simulink model "busCreators01volt"  (R2025b)
settings: Solver=VariableStepAuto  StartTime=0.0  StopTime=10.0  RelTol=1e-3
settings Model: Creator=gdudgeon  LastModifiedBy=gdudgeon
settings RTWCC: GPUComputeCapability=3.5

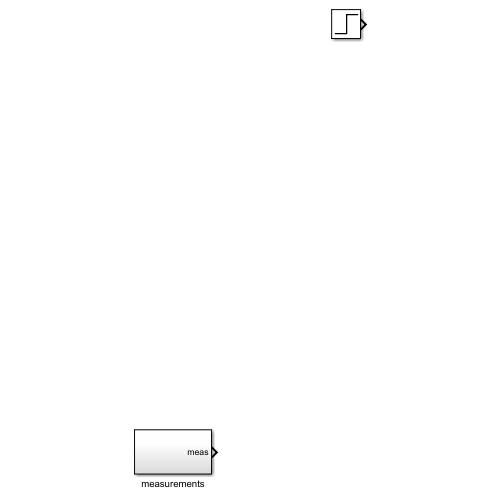
[thumbnail: Simulink's stored preview of the top-level diagram]
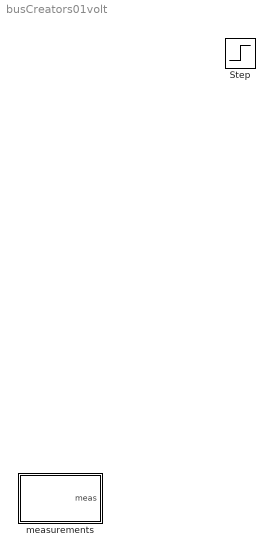
== system busCreators01volt ==
  Step : Step  SampleTime=0
  measurements : Subsystem

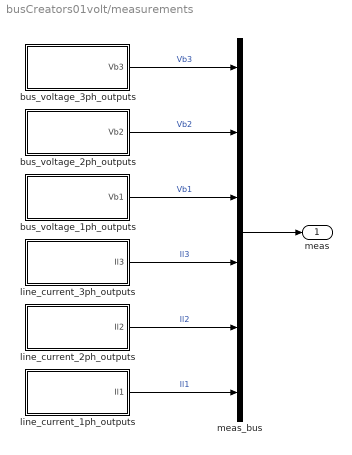
== system busCreators01volt/measurements ==
  bus_voltage_1ph_outputs : Subsystem
  bus_voltage_2ph_outputs : Subsystem
  bus_voltage_3ph_outputs : Subsystem
  line_current_1ph_outputs : Subsystem
  line_current_2ph_outputs : Subsystem
  line_current_3ph_outputs : Subsystem
  meas_bus : BusCreator  Inputs=6
  meas : Outport
  wires:
  line_current_1ph_outputs/1(Il1) -> meas_bus/6  "Il1"
  line_current_2ph_outputs/1(Il2) -> meas_bus/5  "Il2"
  line_current_3ph_outputs/1(Il3) -> meas_bus/4  "Il3"
  meas_bus/1 -> meas/1
  bus_voltage_2ph_outputs/1(Vb2) -> meas_bus/2  "Vb2"
  bus_voltage_3ph_outputs/1(Vb3) -> meas_bus/1  "Vb3"
  bus_voltage_1ph_outputs/1(Vb1) -> meas_bus/3  "Vb1"

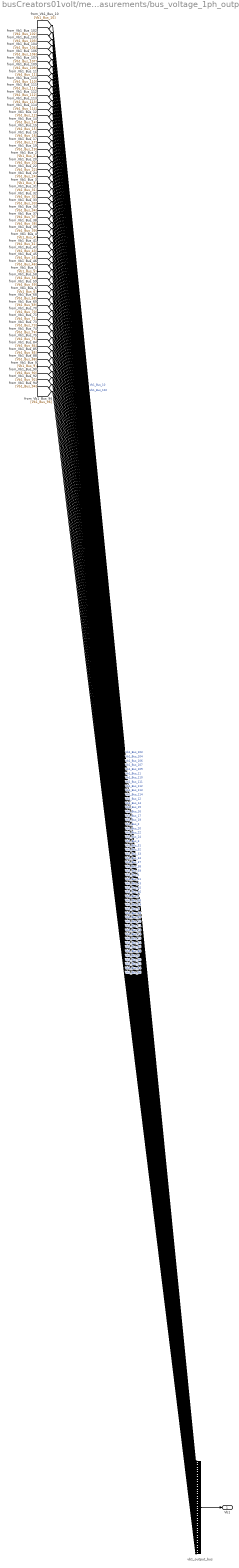
== system busCreators01volt/measurements/bus_voltage_1ph_outputs ==
  vb1_output_bus : BusCreator  Inputs=55
  Vb1 : Outport  OutDataTypeStr=Bus: n1_slBus3  VectorParamsAs1DForOutWhenUnconnected=off
  wires:
  [Vb1_Bus_96] -> vb1_output_bus/55  "Vb1_Bus_96"
  [Vb1_Bus_94] -> vb1_output_bus/54  "Vb1_Bus_94"
  [Vb1_Bus_92] -> vb1_output_bus/53  "Vb1_Bus_92"
  [Vb1_Bus_90] -> vb1_output_bus/52  "Vb1_Bus_90"
  [Vb1_Bus_9] -> vb1_output_bus/51  "Vb1_Bus_9"
  [Vb1_Bus_88] -> vb1_output_bus/50  "Vb1_Bus_88"
  [Vb1_Bus_85] -> vb1_output_bus/49  "Vb1_Bus_85"
  [Vb1_Bus_84] -> vb1_output_bus/48  "Vb1_Bus_84"
  [Vb1_Bus_75] -> vb1_output_bus/47  "Vb1_Bus_75"
  [Vb1_Bus_74] -> vb1_output_bus/46  "Vb1_Bus_74"
  [Vb1_Bus_73] -> vb1_output_bus/45  "Vb1_Bus_73"
  [Vb1_Bus_71] -> vb1_output_bus/44  "Vb1_Bus_71"
  [Vb1_Bus_70] -> vb1_output_bus/43  "Vb1_Bus_70"
  [Vb1_Bus_69] -> vb1_output_bus/42  "Vb1_Bus_69"
  [Vb1_Bus_68] -> vb1_output_bus/41  "Vb1_Bus_68"
  [Vb1_Bus_6] -> vb1_output_bus/40  "Vb1_Bus_6"
  [Vb1_Bus_59] -> vb1_output_bus/39  "Vb1_Bus_59"
  [Vb1_Bus_58] -> vb1_output_bus/38  "Vb1_Bus_58"
  [Vb1_Bus_5] -> vb1_output_bus/37  "Vb1_Bus_5"
  [Vb1_Bus_46] -> vb1_output_bus/36  "Vb1_Bus_46"
  [Vb1_Bus_45] -> vb1_output_bus/35  "Vb1_Bus_45"
  [Vb1_Bus_43] -> vb1_output_bus/34  "Vb1_Bus_43"
  [Vb1_Bus_41] -> vb1_output_bus/33  "Vb1_Bus_41"
  [Vb1_Bus_4] -> vb1_output_bus/32  "Vb1_Bus_4"
  [Vb1_Bus_39] -> vb1_output_bus/31  "Vb1_Bus_39"
  [Vb1_Bus_38] -> vb1_output_bus/30  "Vb1_Bus_38"
  [Vb1_Bus_37] -> vb1_output_bus/29  "Vb1_Bus_37"
  [Vb1_Bus_34] -> vb1_output_bus/28  "Vb1_Bus_34"
  [Vb1_Bus_33] -> vb1_output_bus/27  "Vb1_Bus_33"
  [Vb1_Bus_32] -> vb1_output_bus/26  "Vb1_Bus_32"
  [Vb1_Bus_31] -> vb1_output_bus/25  "Vb1_Bus_31"
  [Vb1_Bus_3] -> vb1_output_bus/24  "Vb1_Bus_3"
  [Vb1_Bus_24] -> vb1_output_bus/23  "Vb1_Bus_24"
  [Vb1_Bus_22] -> vb1_output_bus/22  "Vb1_Bus_22"
  [Vb1_Bus_20] -> vb1_output_bus/21  "Vb1_Bus_20"
  [Vb1_Bus_2] -> vb1_output_bus/20  "Vb1_Bus_2"
  [Vb1_Bus_19] -> vb1_output_bus/19  "Vb1_Bus_19"
  [Vb1_Bus_17] -> vb1_output_bus/18  "Vb1_Bus_17"
  [Vb1_Bus_16] -> vb1_output_bus/17  "Vb1_Bus_16"
  [Vb1_Bus_15] -> vb1_output_bus/16  "Vb1_Bus_15"
  [Vb1_Bus_14] -> vb1_output_bus/15  "Vb1_Bus_14"
  [Vb1_Bus_12] -> vb1_output_bus/14  "Vb1_Bus_12"
  [Vb1_Bus_114] -> vb1_output_bus/13  "Vb1_Bus_114"
  [Vb1_Bus_113] -> vb1_output_bus/12  "Vb1_Bus_113"
  [Vb1_Bus_112] -> vb1_output_bus/11  "Vb1_Bus_112"
  [Vb1_Bus_111] -> vb1_output_bus/10  "Vb1_Bus_111"
  [Vb1_Bus_110] -> vb1_output_bus/9  "Vb1_Bus_110"
  [Vb1_Bus_11] -> vb1_output_bus/8  "Vb1_Bus_11"
  [Vb1_Bus_109] -> vb1_output_bus/7  "Vb1_Bus_109"
  [Vb1_Bus_107] -> vb1_output_bus/6  "Vb1_Bus_107"
  [Vb1_Bus_106] -> vb1_output_bus/5  "Vb1_Bus_106"
  [Vb1_Bus_104] -> vb1_output_bus/4  "Vb1_Bus_104"
  [Vb1_Bus_103] -> vb1_output_bus/3  "Vb1_Bus_103"
  [Vb1_Bus_102] -> vb1_output_bus/2  "Vb1_Bus_102"
  [Vb1_Bus_10] -> vb1_output_bus/1  "Vb1_Bus_10"
  vb1_output_bus/1 -> Vb1/1

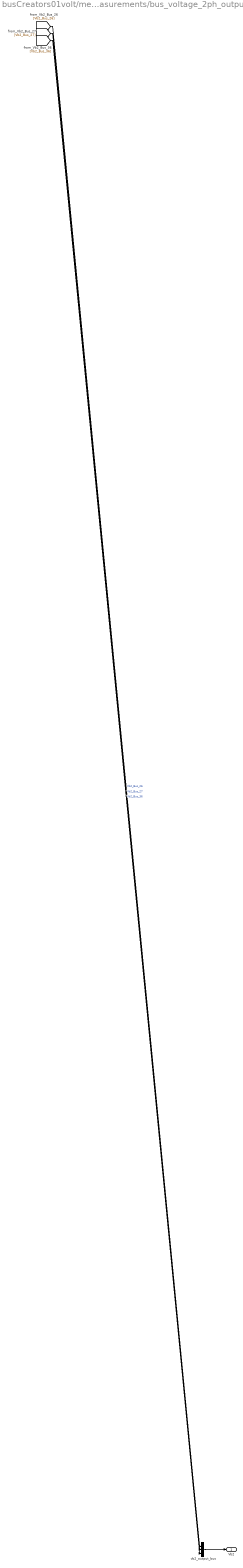
== system busCreators01volt/measurements/bus_voltage_2ph_outputs ==
  vb2_output_bus : BusCreator  Inputs=3
  Vb2 : Outport  OutDataTypeStr=Bus: n1_slBus2  VectorParamsAs1DForOutWhenUnconnected=off
  wires:
  [Vb2_Bus_36] -> vb2_output_bus/3  "Vb2_Bus_36"
  [Vb2_Bus_27] -> vb2_output_bus/2  "Vb2_Bus_27"
  [Vb2_Bus_26] -> vb2_output_bus/1  "Vb2_Bus_26"
  vb2_output_bus/1 -> Vb2/1

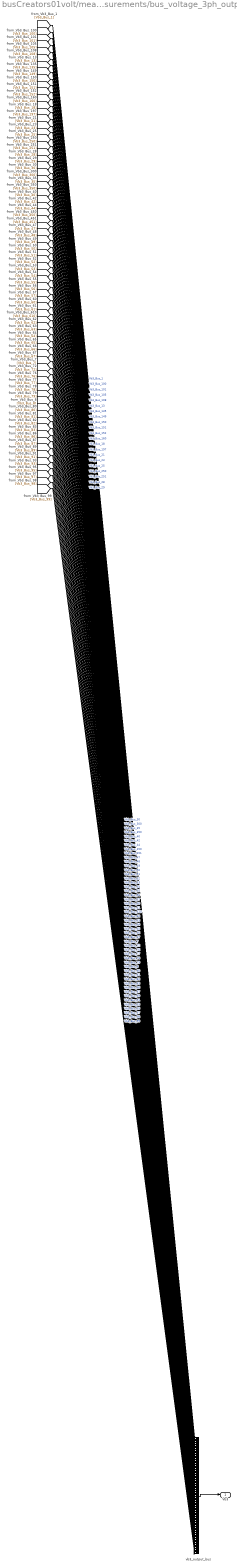
== system busCreators01volt/measurements/bus_voltage_3ph_outputs ==
  vb3_output_bus : BusCreator  Inputs=70
  Vb3 : Outport  OutDataTypeStr=Bus: n1_slBus1  VectorParamsAs1DForOutWhenUnconnected=off
  wires:
  [Vb3_Bus_99] -> vb3_output_bus/70  "Vb3_Bus_99"
  [Vb3_Bus_98] -> vb3_output_bus/69  "Vb3_Bus_98"
  [Vb3_Bus_97] -> vb3_output_bus/68  "Vb3_Bus_97"
  [Vb3_Bus_95] -> vb3_output_bus/67  "Vb3_Bus_95"
  [Vb3_Bus_93] -> vb3_output_bus/66  "Vb3_Bus_93"
  [Vb3_Bus_91] -> vb3_output_bus/65  "Vb3_Bus_91"
  [Vb3_Bus_89] -> vb3_output_bus/64  "Vb3_Bus_89"
  [Vb3_Bus_87] -> vb3_output_bus/63  "Vb3_Bus_87"
  [Vb3_Bus_86] -> vb3_output_bus/62  "Vb3_Bus_86"
  [Vb3_Bus_83] -> vb3_output_bus/61  "Vb3_Bus_83"
  [Vb3_Bus_82] -> vb3_output_bus/60  "Vb3_Bus_82"
  [Vb3_Bus_81] -> vb3_output_bus/59  "Vb3_Bus_81"
  [Vb3_Bus_80] -> vb3_output_bus/58  "Vb3_Bus_80"
  [Vb3_Bus_8] -> vb3_output_bus/57  "Vb3_Bus_8"
  [Vb3_Bus_79] -> vb3_output_bus/56  "Vb3_Bus_79"
  [Vb3_Bus_78] -> vb3_output_bus/55  "Vb3_Bus_78"
  [Vb3_Bus_77] -> vb3_output_bus/54  "Vb3_Bus_77"
  [Vb3_Bus_76] -> vb3_output_bus/53  "Vb3_Bus_76"
  [Vb3_Bus_72] -> vb3_output_bus/52  "Vb3_Bus_72"
  [Vb3_Bus_7] -> vb3_output_bus/51  "Vb3_Bus_7"
  [Vb3_Bus_67] -> vb3_output_bus/50  "Vb3_Bus_67"
  [Vb3_Bus_66] -> vb3_output_bus/49  "Vb3_Bus_66"
  [Vb3_Bus_65] -> vb3_output_bus/48  "Vb3_Bus_65"
  [Vb3_Bus_64] -> vb3_output_bus/47  "Vb3_Bus_64"
  [Vb3_Bus_63] -> vb3_output_bus/46  "Vb3_Bus_63"
  [Vb3_Bus_62] -> vb3_output_bus/45  "Vb3_Bus_62"
  [Vb3_Bus_610] -> vb3_output_bus/44  "Vb3_Bus_610"
  [Vb3_Bus_61] -> vb3_output_bus/43  "Vb3_Bus_61"
  [Vb3_Bus_60] -> vb3_output_bus/42  "Vb3_Bus_60"
  [Vb3_Bus_57] -> vb3_output_bus/41  "Vb3_Bus_57"
  [Vb3_Bus_56] -> vb3_output_bus/40  "Vb3_Bus_56"
  [Vb3_Bus_55] -> vb3_output_bus/39  "Vb3_Bus_55"
  [Vb3_Bus_54] -> vb3_output_bus/38  "Vb3_Bus_54"
  [Vb3_Bus_53] -> vb3_output_bus/37  "Vb3_Bus_53"
  [Vb3_Bus_52] -> vb3_output_bus/36  "Vb3_Bus_52"
  [Vb3_Bus_51] -> vb3_output_bus/35  "Vb3_Bus_51"
  [Vb3_Bus_50] -> vb3_output_bus/34  "Vb3_Bus_50"
  [Vb3_Bus_49] -> vb3_output_bus/33  "Vb3_Bus_49"
  [Vb3_Bus_48] -> vb3_output_bus/32  "Vb3_Bus_48"
  [Vb3_Bus_47] -> vb3_output_bus/31  "Vb3_Bus_47"
  [Vb3_Bus_451] -> vb3_output_bus/30  "Vb3_Bus_451"
  [Vb3_Bus_450] -> vb3_output_bus/29  "Vb3_Bus_450"
  [Vb3_Bus_44] -> vb3_output_bus/28  "Vb3_Bus_44"
  [Vb3_Bus_42] -> vb3_output_bus/27  "Vb3_Bus_42"
  [Vb3_Bus_40] -> vb3_output_bus/26  "Vb3_Bus_40"
  [Vb3_Bus_350] -> vb3_output_bus/25  "Vb3_Bus_350"
  [Vb3_Bus_35] -> vb3_output_bus/24  "Vb3_Bus_35"
  [Vb3_Bus_300] -> vb3_output_bus/23  "Vb3_Bus_300"
  [Vb3_Bus_30] -> vb3_output_bus/22  "Vb3_Bus_30"
  [Vb3_Bus_29] -> vb3_output_bus/21  "Vb3_Bus_29"
  [Vb3_Bus_28] -> vb3_output_bus/20  "Vb3_Bus_28"
  [Vb3_Bus_251] -> vb3_output_bus/19  "Vb3_Bus_251"
  [Vb3_Bus_250] -> vb3_output_bus/18  "Vb3_Bus_250"
  [Vb3_Bus_25] -> vb3_output_bus/17  "Vb3_Bus_25"
  [Vb3_Bus_23] -> vb3_output_bus/16  "Vb3_Bus_23"
  [Vb3_Bus_21] -> vb3_output_bus/15  "Vb3_Bus_21"
  [Vb3_Bus_197] -> vb3_output_bus/14  "Vb3_Bus_197"
  [Vb3_Bus_18] -> vb3_output_bus/13  "Vb3_Bus_18"
  [Vb3_Bus_160] -> vb3_output_bus/12  "Vb3_Bus_160"
  [Vb3_Bus_152] -> vb3_output_bus/11  "Vb3_Bus_152"
  [Vb3_Bus_151] -> vb3_output_bus/10  "Vb3_Bus_151"
  [Vb3_Bus_150] -> vb3_output_bus/9  "Vb3_Bus_150"
  [Vb3_Bus_149] -> vb3_output_bus/8  "Vb3_Bus_149"
  [Vb3_Bus_135] -> vb3_output_bus/7  "Vb3_Bus_135"
  [Vb3_Bus_13] -> vb3_output_bus/6  "Vb3_Bus_13"
  [Vb3_Bus_108] -> vb3_output_bus/5  "Vb3_Bus_108"
  [Vb3_Bus_105] -> vb3_output_bus/4  "Vb3_Bus_105"
  [Vb3_Bus_101] -> vb3_output_bus/3  "Vb3_Bus_101"
  [Vb3_Bus_100] -> vb3_output_bus/2  "Vb3_Bus_100"
  [Vb3_Bus_1] -> vb3_output_bus/1  "Vb3_Bus_1"
  vb3_output_bus/1 -> Vb3/1

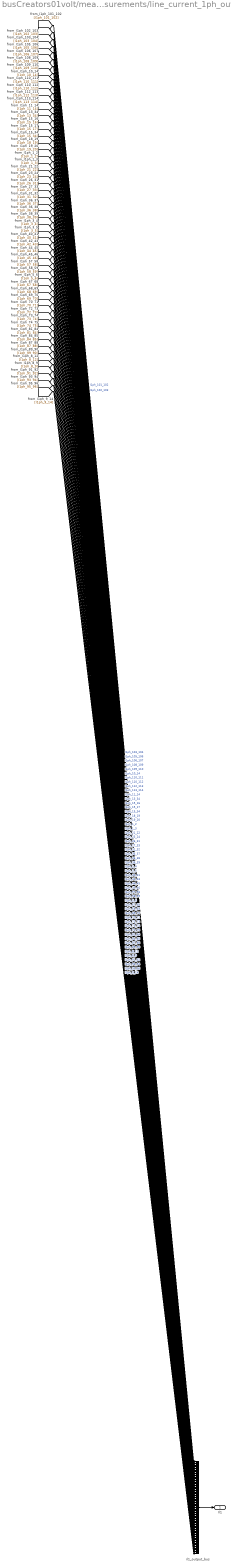
== system busCreators01volt/measurements/line_current_1ph_outputs ==
  il1_output_bus : BusCreator  Inputs=55
  Il1 : Outport  OutDataTypeStr=Bus: n1_slBus6  VectorParamsAs1DForOutWhenUnconnected=off
  wires:
  [I1ph_9_14] -> il1_output_bus/55  "I1ph_9_14"
  [I1ph_95_96] -> il1_output_bus/54  "I1ph_95_96"
  [I1ph_93_94] -> il1_output_bus/53  "I1ph_93_94"
  [I1ph_91_92] -> il1_output_bus/52  "I1ph_91_92"
  [I1ph_8_9] -> il1_output_bus/51  "I1ph_8_9"
  [I1ph_8_12] -> il1_output_bus/50  "I1ph_8_12"
  [I1ph_89_90] -> il1_output_bus/49  "I1ph_89_90"
  [I1ph_87_88] -> il1_output_bus/48  "I1ph_87_88"
  [I1ph_84_85] -> il1_output_bus/47  "I1ph_84_85"
  [I1ph_81_84] -> il1_output_bus/46  "I1ph_81_84"
  [I1ph_74_75] -> il1_output_bus/45  "I1ph_74_75"
  [I1ph_73_74] -> il1_output_bus/44  "I1ph_73_74"
  [I1ph_72_73] -> il1_output_bus/43  "I1ph_72_73"
  [I1ph_70_71] -> il1_output_bus/42  "I1ph_70_71"
  [I1ph_69_70] -> il1_output_bus/41  "I1ph_69_70"
  [I1ph_68_69] -> il1_output_bus/40  "I1ph_68_69"
  [I1ph_67_68] -> il1_output_bus/39  "I1ph_67_68"
  [I1ph_5_6] -> il1_output_bus/38  "I1ph_5_6"
  [I1ph_58_59] -> il1_output_bus/37  "I1ph_58_59"
  [I1ph_57_58] -> il1_output_bus/36  "I1ph_57_58"
  [I1ph_45_46] -> il1_output_bus/35  "I1ph_45_46"
  [I1ph_44_45] -> il1_output_bus/34  "I1ph_44_45"
  [I1ph_42_43] -> il1_output_bus/33  "I1ph_42_43"
  [I1ph_40_41] -> il1_output_bus/32  "I1ph_40_41"
  [I1ph_3_5] -> il1_output_bus/31  "I1ph_3_5"
  [I1ph_3_4] -> il1_output_bus/30  "I1ph_3_4"
  [I1ph_38_39] -> il1_output_bus/29  "I1ph_38_39"
  [I1ph_36_38] -> il1_output_bus/28  "I1ph_36_38"
  [I1ph_36_37] -> il1_output_bus/27  "I1ph_36_37"
  [I1ph_31_32] -> il1_output_bus/26  "I1ph_31_32"
  [I1ph_27_33] -> il1_output_bus/25  "I1ph_27_33"
  [I1ph_26_31] -> il1_output_bus/24  "I1ph_26_31"
  [I1ph_23_24] -> il1_output_bus/23  "I1ph_23_24"
  [I1ph_21_22] -> il1_output_bus/22  "I1ph_21_22"
  [I1ph_1_3] -> il1_output_bus/21  "I1ph_1_3"
  [I1ph_1_2] -> il1_output_bus/20  "I1ph_1_2"
  [I1ph_19_20] -> il1_output_bus/19  "I1ph_19_20"
  [I1ph_18_19] -> il1_output_bus/18  "I1ph_18_19"
  [I1ph_15_34] -> il1_output_bus/17  "I1ph_15_34"
  [I1ph_15_17] -> il1_output_bus/16  "I1ph_15_17"
  [I1ph_15_16] -> il1_output_bus/15  "I1ph_15_16"
  [I1ph_13_34] -> il1_output_bus/14  "I1ph_13_34"
  [I1ph_11_14] -> il1_output_bus/13  "I1ph_11_14"
  [I1ph_113_114] -> il1_output_bus/12  "I1ph_113_114"
  [I1ph_112_113] -> il1_output_bus/11  "I1ph_112_113"
  [I1ph_110_112] -> il1_output_bus/10  "I1ph_110_112"
  [I1ph_110_111] -> il1_output_bus/9  "I1ph_110_111"
  [I1ph_10_14] -> il1_output_bus/8  "I1ph_10_14"
  [I1ph_109_110] -> il1_output_bus/7  "I1ph_109_110"
  [I1ph_108_109] -> il1_output_bus/6  "I1ph_108_109"
  [I1ph_106_107] -> il1_output_bus/5  "I1ph_106_107"
  [I1ph_105_106] -> il1_output_bus/4  "I1ph_105_106"
  [I1ph_103_104] -> il1_output_bus/3  "I1ph_103_104"
  [I1ph_102_103] -> il1_output_bus/2  "I1ph_102_103"
  [I1ph_101_102] -> il1_output_bus/1  "I1ph_101_102"
  il1_output_bus/1 -> Il1/1

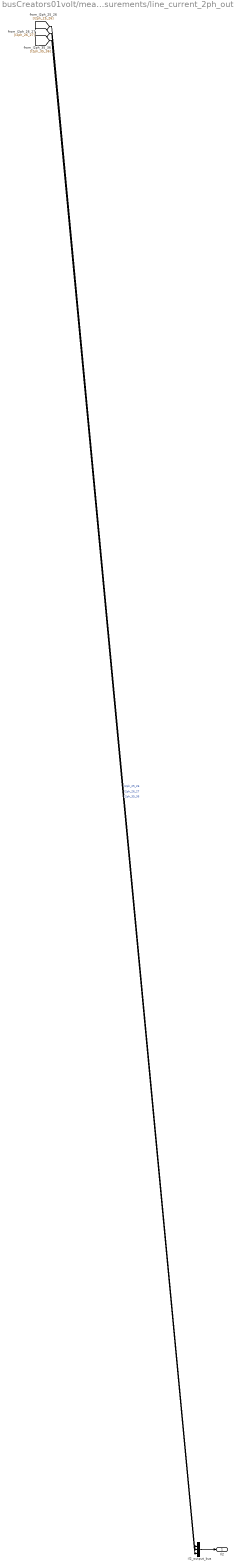
== system busCreators01volt/measurements/line_current_2ph_outputs ==
  il2_output_bus : BusCreator  Inputs=3
  Il2 : Outport  OutDataTypeStr=Bus: n1_slBus5  VectorParamsAs1DForOutWhenUnconnected=off
  wires:
  [I2ph_35_36] -> il2_output_bus/3  "I2ph_35_36"
  [I2ph_26_27] -> il2_output_bus/2  "I2ph_26_27"
  [I2ph_25_26] -> il2_output_bus/1  "I2ph_25_26"
  il2_output_bus/1 -> Il2/1

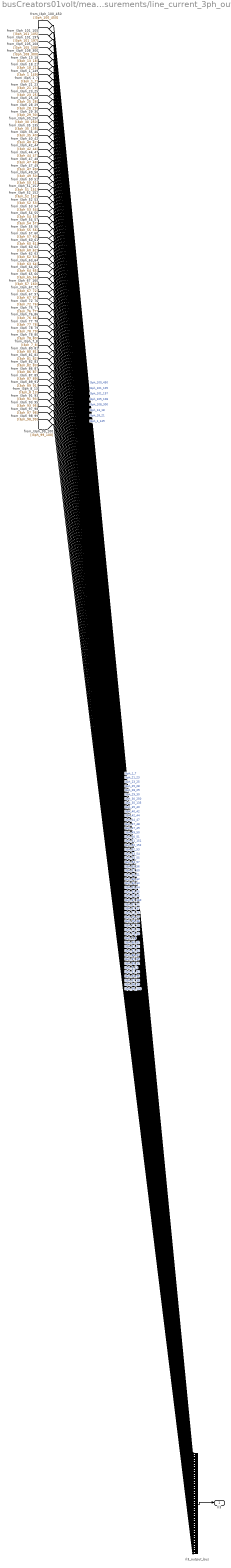
== system busCreators01volt/measurements/line_current_3ph_outputs ==
  il3_output_bus : BusCreator  Inputs=60
  Il3 : Outport  OutDataTypeStr=Bus: n1_slBus4  VectorParamsAs1DForOutWhenUnconnected=off
  wires:
  [I3ph_99_100] -> il3_output_bus/60  "I3ph_99_100"
  [I3ph_98_99] -> il3_output_bus/59  "I3ph_98_99"
  [I3ph_97_98] -> il3_output_bus/58  "I3ph_97_98"
  [I3ph_93_95] -> il3_output_bus/57  "I3ph_93_95"
  [I3ph_91_93] -> il3_output_bus/56  "I3ph_91_93"
  [I3ph_8_13] -> il3_output_bus/55  "I3ph_8_13"
  [I3ph_89_91] -> il3_output_bus/54  "I3ph_89_91"
  [I3ph_87_89] -> il3_output_bus/53  "I3ph_87_89"
  [I3ph_86_87] -> il3_output_bus/52  "I3ph_86_87"
  [I3ph_82_83] -> il3_output_bus/51  "I3ph_82_83"
  [I3ph_81_82] -> il3_output_bus/50  "I3ph_81_82"
  [I3ph_80_81] -> il3_output_bus/49  "I3ph_80_81"
  [I3ph_7_8] -> il3_output_bus/48  "I3ph_7_8"
  [I3ph_78_80] -> il3_output_bus/47  "I3ph_78_80"
  [I3ph_78_79] -> il3_output_bus/46  "I3ph_78_79"
  [I3ph_77_78] -> il3_output_bus/45  "I3ph_77_78"
  [I3ph_76_86] -> il3_output_bus/44  "I3ph_76_86"
  [I3ph_76_77] -> il3_output_bus/43  "I3ph_76_77"
  [I3ph_72_76] -> il3_output_bus/42  "I3ph_72_76"
  [I3ph_67_97] -> il3_output_bus/41  "I3ph_67_97"
  [I3ph_67_72] -> il3_output_bus/40  "I3ph_67_72"
  [I3ph_67_160] -> il3_output_bus/39  "I3ph_67_160"
  [I3ph_65_66] -> il3_output_bus/38  "I3ph_65_66"
  [I3ph_64_65] -> il3_output_bus/37  "I3ph_64_65"
  [I3ph_63_64] -> il3_output_bus/36  "I3ph_63_64"
  [I3ph_62_63] -> il3_output_bus/35  "I3ph_62_63"
  [I3ph_60_62] -> il3_output_bus/34  "I3ph_60_62"
  [I3ph_60_61] -> il3_output_bus/33  "I3ph_60_61"
  [I3ph_57_60] -> il3_output_bus/32  "I3ph_57_60"
  [I3ph_55_56] -> il3_output_bus/31  "I3ph_55_56"
  [I3ph_54_57] -> il3_output_bus/30  "I3ph_54_57"
  [I3ph_54_55] -> il3_output_bus/29  "I3ph_54_55"
  [I3ph_53_54] -> il3_output_bus/28  "I3ph_53_54"
  [I3ph_52_53] -> il3_output_bus/27  "I3ph_52_53"
  [I3ph_52_152] -> il3_output_bus/26  "I3ph_52_152"
  [I3ph_51_151] -> il3_output_bus/25  "I3ph_51_151"
  [I3ph_50_51] -> il3_output_bus/24  "I3ph_50_51"
  [I3ph_49_50] -> il3_output_bus/23  "I3ph_49_50"
  [I3ph_47_49] -> il3_output_bus/22  "I3ph_47_49"
  [I3ph_47_48] -> il3_output_bus/21  "I3ph_47_48"
  [I3ph_44_47] -> il3_output_bus/20  "I3ph_44_47"
  [I3ph_42_44] -> il3_output_bus/19  "I3ph_42_44"
  [I3ph_40_42] -> il3_output_bus/18  "I3ph_40_42"
  [I3ph_35_40] -> il3_output_bus/17  "I3ph_35_40"
  [I3ph_35_135] -> il3_output_bus/16  "I3ph_35_135"
  [I3ph_30_250] -> il3_output_bus/15  "I3ph_30_250"
  [I3ph_29_30] -> il3_output_bus/14  "I3ph_29_30"
  [I3ph_28_29] -> il3_output_bus/13  "I3ph_28_29"
  [I3ph_25_28] -> il3_output_bus/12  "I3ph_25_28"
  [I3ph_23_25] -> il3_output_bus/11  "I3ph_23_25"
  [I3ph_21_23] -> il3_output_bus/10  "I3ph_21_23"
  [I3ph_1_7] -> il3_output_bus/9  "I3ph_1_7"
  [I3ph_1_149] -> il3_output_bus/8  "I3ph_1_149"
  [I3ph_18_21] -> il3_output_bus/7  "I3ph_18_21"
  [I3ph_13_18] -> il3_output_bus/6  "I3ph_13_18"
  [I3ph_108_300] -> il3_output_bus/5  "I3ph_108_300"
  [I3ph_105_108] -> il3_output_bus/4  "I3ph_105_108"
  [I3ph_101_197] -> il3_output_bus/3  "I3ph_101_197"
  [I3ph_101_105] -> il3_output_bus/2  "I3ph_101_105"
  [I3ph_100_450] -> il3_output_bus/1  "I3ph_100_450"
  il3_output_bus/1 -> Il3/1
